simulink model "doe_model_standalone"  (R2023a)
settings: Solver=VariableStepAuto  StartTime=0.0  StopTime=10.0  RelTol=1e-3
PreLoadFcn:
  | run('stack_subsystem_supply_bus_definitions.m')
  | addpath(genpath(fullfile('..','p10_doe_basic_files')))
undefined symbols (not defined in the file): dewpoint_temperature_degC, h2_molar_concentration, inlet_flow_lpmin, inlet_pressure_barg, inlet_temperature_degC, stoichiometry
settings Model: Creator=stefan.notter  LastModifiedBy=stefan.notter

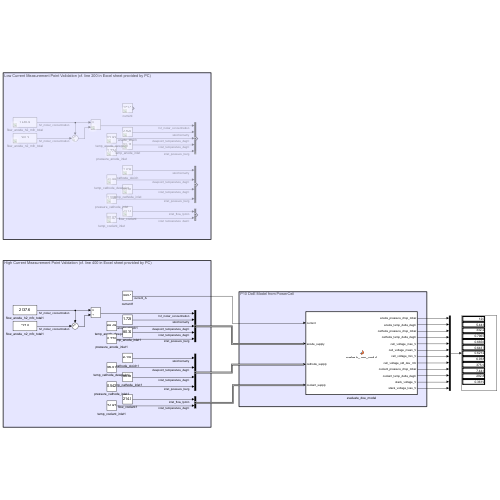
[thumbnail: Simulink's stored preview of the top-level diagram]
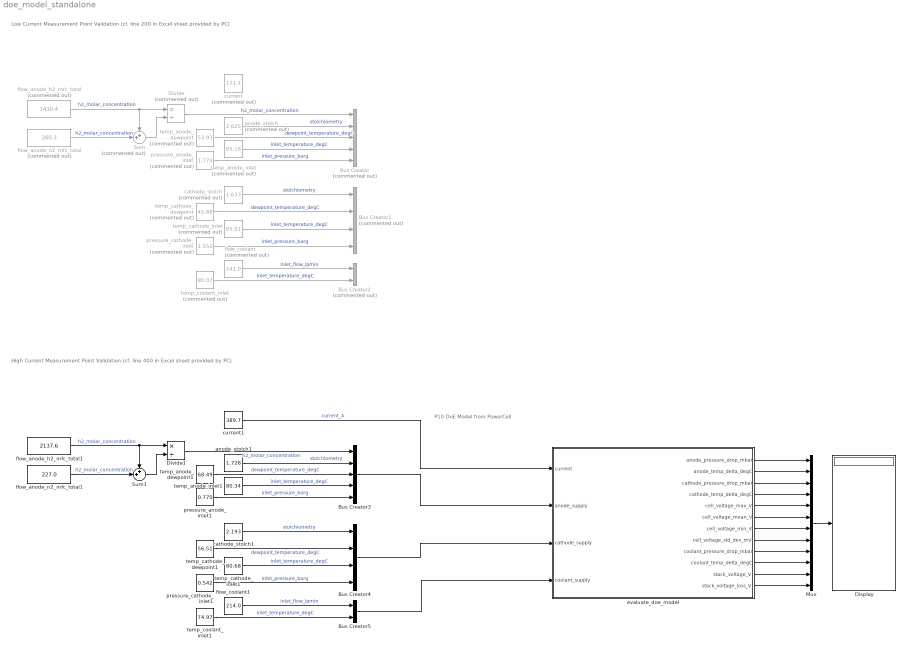
== system doe_model_standalone ==
  note: Low Current Measurement Point Validation (cf. line 200 in Excel sheet provided by PC)
  note: P10 DoE Model from PowerCell
  note: High Current Measurement Point Validation (cf. line 400 in Excel sheet provided by PC)
  Bus Creator : BusCreator  Commented=on  Inputs=h2_molar_concentration,stoichiometry,dewpoint_temperature_degC,inlet_temperature_degC,inlet_pressure_barg  OutDataTypeStr=Bus: anode_supply
  Bus Creator1 : BusCreator  Commented=on  Inputs=stoichiometry,dewpoint_temperature_degC,inlet_temperature_degC,inlet_pressure_barg  OutDataTypeStr=Bus: cathode_supply
  Bus Creator2 : BusCreator  Commented=on  Inputs=inlet_flow_lpmin,inlet_temperature_degC  OutDataTypeStr=Bus: coolant_supply
  Bus Creator3 : BusCreator  Inputs=h2_molar_concentration,stoichiometry,dewpoint_temperature_degC,inlet_temperature_degC,inlet_pressure_barg  OutDataTypeStr=Bus: anode_supply
  Bus Creator4 : BusCreator  Inputs=stoichiometry,dewpoint_temperature_degC,inlet_temperature_degC,inlet_pressure_barg  OutDataTypeStr=Bus: cathode_supply
  Bus Creator5 : BusCreator  Inputs=inlet_flow_lpmin,inlet_temperature_degC  OutDataTypeStr=Bus: coolant_supply
  Display : Display
  Divide : Product  Commented=on  Inputs=*/
  Divide1 : Product  Inputs=*/
  Mux : Mux  Inputs=12
  Sum : Sum  Commented=on  Inputs=++|
  Sum1 : Sum  Inputs=++|
  anode_stoich : Constant  Commented=on  Value=2.625
  anode_stoich1 : Constant  Value=1.728
  cathode_stoich : Constant  Commented=on  Value=1.633
  cathode_stoich1 : Constant  Value=2.193
  current : Constant  Commented=on  Value=171.7
  current1 : Constant  Value=389.7
  evaluate_doe_model : MATLAB Function  TreatAsAtomicUnit=on  SystemSampleTime=1
  flow_anode_h2_mfc_total : Constant  Commented=on  Value=1430.4
  flow_anode_h2_mfc_total1 : Constant  Value=2137.6
  flow_anode_n2_mfc_total : Constant  Commented=on  Value=260.3
  flow_anode_n2_mfc_total1 : Constant  Value=227.0
  flow_coolant : Constant  Commented=on  Value=241.0
  flow_coolant1 : Constant  Value=214.0
  pressure_anode_inlet : Constant  Commented=on  Value=1.774
  pressure_anode_inlet1 : Constant  Value=0.770
  pressure_cathode_inlet : Constant  Commented=on  Value=1.550
  pressure_cathode_inlet1 : Constant  Value=0.542
  temp_anode_dewpoint : Constant  Commented=on  Value=53.93
  temp_anode_dewpoint1 : Constant  Value=68.49
  temp_anode_inlet : Constant  Commented=on  Value=85.18
  temp_anode_inlet1 : Constant  Value=80.34
  temp_cathode_dewpoint : Constant  Commented=on  Value=45.88
  temp_cathode_dewpoint1 : Constant  Value=56.51
  temp_cathode_inlet : Constant  Commented=on  Value=85.01
  temp_cathode_inlet1 : Constant  Value=80.68
  temp_coolant_inlet : Constant  Commented=on  Value=80.07
  temp_coolant_inlet1 : Constant  Value=74.97
  wires:
  anode_stoich/1 -> Bus Creator/2  "stoichiometry"
  temp_anode_inlet/1 -> Bus Creator/4  "inlet_temperature_degC"
  flow_coolant/1 -> Bus Creator2/1  "inlet_flow_lpmin"
  Divide/1 -> Bus Creator/1  "h2_molar_concentration"
  cathode_stoich/1 -> Bus Creator1/1  "stoichiometry"
  temp_coolant_inlet/1 -> Bus Creator2/2  "inlet_temperature_degC"
  temp_anode_dewpoint/1 -> Bus Creator/3  "dewpoint_temperature_degC"
  pressure_cathode_inlet/1 -> Bus Creator1/4  "inlet_pressure_barg"
  temp_cathode_inlet/1 -> Bus Creator1/3  "inlet_temperature_degC"
  pressure_anode_inlet/1 -> Bus Creator/5  "inlet_pressure_barg"
  temp_cathode_dewpoint/1 -> Bus Creator1/2  "dewpoint_temperature_degC"
  evaluate_doe_model/1(anode_pressure_drop_mbar) -> Mux/1
  evaluate_doe_model/2(anode_temp_delta_degC) -> Mux/2
  evaluate_doe_model/3(cathode_pressure_drop_mbar) -> Mux/3
  evaluate_doe_model/4(cathode_temp_delta_degC) -> Mux/4
  evaluate_doe_model/5(cell_voltage_max_V) -> Mux/5
  evaluate_doe_model/6(cell_voltage_mean_V) -> Mux/6
  evaluate_doe_model/7(cell_voltage_min_V) -> Mux/7
  evaluate_doe_model/8(cell_voltage_std_dev_mV) -> Mux/8
  evaluate_doe_model/9(coolant_pressure_drop_mbar) -> Mux/9
  evaluate_doe_model/10(coolant_temp_delta_degC) -> Mux/10
  evaluate_doe_model/11(stack_voltage_V) -> Mux/11
  evaluate_doe_model/12(stack_voltage_loss_V) -> Mux/12
  flow_anode_h2_mfc_total/1 -> Sum/1, Divide/1  "h2_molar_concentration"
  flow_anode_n2_mfc_total/1 -> Sum/2  "h2_molar_concentration"
  Sum/1 -> Divide/2
  Divide1/1 -> Bus Creator3/1  "h2_molar_concentration"
  Sum1/1 -> Divide1/2
  temp_cathode_dewpoint1/1 -> Bus Creator4/2  "dewpoint_temperature_degC"
  temp_coolant_inlet1/1 -> Bus Creator5/2  "inlet_temperature_degC"
  pressure_anode_inlet1/1 -> Bus Creator3/5  "inlet_pressure_barg"
  temp_cathode_inlet1/1 -> Bus Creator4/3  "inlet_temperature_degC"
  temp_anode_inlet1/1 -> Bus Creator3/4  "inlet_temperature_degC"
  temp_anode_dewpoint1/1 -> Bus Creator3/3  "dewpoint_temperature_degC"
  cathode_stoich1/1 -> Bus Creator4/1  "stoichiometry"
  flow_coolant1/1 -> Bus Creator5/1  "inlet_flow_lpmin"
  pressure_cathode_inlet1/1 -> Bus Creator4/4  "inlet_pressure_barg"
  flow_anode_h2_mfc_total1/1 -> Sum1/1, Divide1/1  "h2_molar_concentration"
  flow_anode_n2_mfc_total1/1 -> Sum1/2  "h2_molar_concentration"
  anode_stoich1/1 -> Bus Creator3/2  "stoichiometry"
  Bus Creator5/1 -> evaluate_doe_model/4(coolant_supply)
  Bus Creator4/1 -> evaluate_doe_model/3(cathode_supply)
  Bus Creator3/1 -> evaluate_doe_model/2(anode_supply)
  current1/1 -> evaluate_doe_model/1(current)  "current_A"
  Mux/1 -> Display/1

== matlab function doe_model_standalone/evaluate_doe_model ==
  data: current input; anode_pressure_drop_mbar output; anode_temp_delta_degC output; cathode_pressure_drop_mbar output; cathode_temp_delta_degC output; cell_voltage_max_V output; cell_voltage_mean_V output; cell_voltage_min_V output; cell_voltage_std_dev_mV output; coolant_pressure_drop_mbar output; coolant_temp_delta_degC output; stack_voltage_V output; anode_supply input; stack_voltage_loss_V output; cathode_supply input; coolant_supply input
function [anode_pressure_drop_mbar, anode_temp_delta_degC, cathode_pressure_drop_mbar, ...
cathode_temp_delta_degC, cell_voltage_max_V, cell_voltage_mean_V, cell_voltage_min_V, ...
cell_voltage_std_dev_mV, coolant_pressure_drop_mbar, coolant_temp_delta_degC, ...
stack_voltage_V, stack_voltage_loss_V] = evaluate_doe_model(current, anode_supply, cathode_supply, coolant_supply)

% This function calls the .mex files created from PowerCell response
% surface interpolation of DoE data by providing the input arguments: 
% [current, anode_supply, cathode_supply, coolant_supply]. Note that the
% "model is only valid within the range of tested data." For more
% information, see: p10_doe_files\vendor_provision\Stack_Data_Model_Information.pdf

%% exclude .mex files from code generation

coder.extrinsic('get_anode_pressure_drop', 'get_anode_temp_delta', ...
    'get_cathode_pressure_drop', 'get_cathode_temp_delta', 'get_cell_voltage_max', ...
    'get_cell_voltage_mean', 'get_cell_voltage_min', 'get_cell_voltage_std_dev', ...
    'get_coolant_pressure_drop', 'get_coolant_temp_delta', 'get_stack_voltage', ...
    'get_stack_voltage_loss')

%% instantiate .mex file return variables as doubles

anode_pressure_drop_mbar = double(0);
anode_temp_delta_degC = double(0);
cathode_pressure_drop_mbar = double(0);
cathode_temp_delta_degC = double(0);
cell_voltage_max_V = double(0);
cell_voltage_mean_V = double(0);
cell_voltage_min_V = double(0);
cell_voltage_std_dev_mV = double(0);
coolant_pressure_drop_mbar = double(0);
coolant_temp_delta_degC = double(0);
stack_voltage_V = double(0);
stack_voltage_loss_V = double(0);

%% call .mex files created from PowerCell response surface interpolation of DoE data

anode_pressure_drop_mbar = get_anode_pressure_drop(current, ...
    anode_supply.h2_molar_concentration, anode_supply.stoichiometry, anode_supply.dewpoint_temperature_degC, anode_supply.inlet_temperature_degC, anode_supply.inlet_pressure_barg, ...
    cathode_supply.stoichiometry, cathode_supply.dewpoint_temperature_degC, cathode_supply.inlet_temperature_degC, cathode_supply.inlet_pressure_barg, ...
    coolant_supply.inlet_flow_lpmin, coolant_supply.inlet_temperature_degC);
anode_temp_delta_degC = get_anode_temp_delta(current, ...
    anode_supply.h2_molar_concentration, anode_supply.stoichiometry, anode_supply.dewpoint_temperature_degC, anode_supply.inlet_temperature_degC, anode_supply.inlet_pressure_barg, ...
    cathode_supply.stoichiometry, cathode_supply.dewpoint_temperature_degC, cathode_supply.inlet_temperature_degC, cathode_supply.inlet_pressure_barg, ...
    coolant_supply.inlet_flow_lpmin, coolant_supply.inlet_temperature_degC);
cathode_pressure_drop_mbar = get_cathode_pressure_drop(current, ...
    anode_supply.h2_molar_concentration, anode_supply.stoichiometry, anode_supply.dewpoint_temperature_degC, anode_supply.inlet_temperature_degC, anode_supply.inlet_pressure_barg, ...
    cathode_supply.stoichiometry, cathode_supply.dewpoint_temperature_degC, cathode_supply.inlet_temperature_degC, cathode_supply.inlet_pressure_barg, ...
    coolant_supply.inlet_flow_lpmin, coolant_supply.inlet_temperature_degC);
cathode_temp_delta_degC = get_cathode_temp_delta(current, ...
    anode_supply.h2_molar_concentration, anode_supply.stoichiometry, anode_supply.dewpoint_temperature_degC, anode_supply.inlet_temperature_degC, anode_supply.inlet_pressure_barg, ...
    cathode_supply.stoichiometry, cathode_supply.dewpoint_temperature_degC, cathode_supply.inlet_temperature_degC, cathode_supply.inlet_pressure_barg, ...
    coolant_supply.inlet_flow_lpmin, coolant_supply.inlet_temperature_degC);
cell_voltage_max_V = get_cell_voltage_max(current, ...
    anode_supply.h2_molar_concentration, anode_supply.stoichiometry, anode_supply.dewpoint_temperature_degC, anode_supply.inlet_temperature_degC, anode_supply.inlet_pressure_barg, ...
    cathode_supply.stoichiometry, cathode_supply.dewpoint_temperature_degC, cathode_supply.inlet_temperature_degC, cathode_supply.inlet_pressure_barg, ...
    coolant_supply.inlet_flow_lpmin, coolant_supply.inlet_temperature_degC);
cell_voltage_mean_V = get_cell_voltage_mean(current, ...
    anode_supply.h2_molar_concentration, anode_supply.stoichiometry, anode_supply.dewpoint_temperature_degC, anode_supply.inlet_temperature_degC, anode_supply.inlet_pressure_barg, ...
    cathode_supply.stoichiometry, cathode_supply.dewpoint_temperature_degC, cathode_supply.inlet_temperature_degC, cathode_supply.inlet_pressure_barg, ...
    coolant_supply.inlet_flow_lpmin, coolant_supply.inlet_temperature_degC);
cell_voltage_min_V = get_cell_voltage_min(current, ...
    anode_supply.h2_molar_concentration, anode_supply.stoichiometry, anode_supply.dewpoint_temperature_degC, anode_supply.inlet_temperature_degC, anode_supply.inlet_pressure_barg, ...
    cathode_supply.stoichiometry, cathode_supply.dewpoint_temperature_degC, cathode_supply.inlet_temperature_degC, cathode_supply.inlet_pressure_barg, ...
    coolant_supply.inlet_flow_lpmin, coolant_supply.inlet_temperature_degC);
cell_voltage_std_dev_mV = get_cell_voltage_std_dev(current, ...
    anode_supply.h2_molar_concentration, anode_supply.stoichiometry, anode_supply.dewpoint_temperature_degC, anode_supply.inlet_temperature_degC, anode_supply.inlet_pressure_barg, ...
    cathode_supply.stoichiometry, cathode_supply.dewpoint_temperature_degC, cathode_supply.inlet_temperature_degC, cathode_supply.inlet_pressure_barg, ...
    coolant_supply.inlet_flow_lpmin, coolant_supply.inlet_temperature_degC);
coolant_pressure_drop_mbar = get_coolant_pressure_drop(current, ...
    anode_supply.h2_molar_concentration, anode_supply.stoichiometry, anode_supply.dewpoint_temperature_degC, anode_supply.inlet_temperature_degC, anode_supply.inlet_pressure_barg, ...
    cathode_supply.stoichiometry, cathode_supply.dewpoint_temperature_degC, cathode_supply.inlet_temperature_degC, cathode_supply.inlet_pressure_barg, ...
    coolant_supply.inlet_flow_lpmin, coolant_supply.inlet_temperature_degC);
coolant_temp_delta_degC = get_coolant_temp_delta(current, ...
    anode_supply.h2_molar_concentration, anode_supply.stoichiometry, anode_supply.dewpoint_temperature_degC, anode_supply.inlet_temperature_degC, anode_supply.inlet_pressure_barg, ...
    cathode_supply.stoichiometry, cathode_supply.dewpoint_temperature_degC, cathode_supply.inlet_temperature_degC, cathode_supply.inlet_pressure_barg, ...
    coolant_supply.inlet_flow_lpmin, coolant_supply.inlet_temperature_degC);
stack_voltage_V = get_stack_voltage(current, ...
    anode_supply.h2_molar_concentration, anode_supply.stoichiometry, anode_supply.dewpoint_temperature_degC, anode_supply.inlet_temperature_degC, anode_supply.inlet_pressure_barg, ...
    cathode_supply.stoichiometry, cathode_supply.dewpoint_temperature_degC, cathode_supply.inlet_temperature_degC, cathode_supply.inlet_pressure_barg, ...
    coolant_supply.inlet_flow_lpmin, coolant_supply.inlet_temperature_degC);
stack_voltage_loss_V = get_stack_voltage_loss(current, ...
    anode_supply.h2_molar_concentration, anode_supply.stoichiometry, anode_supply.dewpoint_temperature_degC, anode_supply.inlet_temperature_degC, anode_supply.inlet_pressure_barg, ...
    cathode_supply.stoichiometry, cathode_supply.dewpoint_temperature_degC, cathode_supply.inlet_temperature_degC, cathode_supply.inlet_pressure_barg, ...
    coolant_supply.inlet_flow_lpmin, coolant_supply.inlet_temperature_degC);
